simulink model "cosmic_ray_system"  (R2019a)
settings: Solver=VariableStepAuto  StartTime=0.0  StopTime=1000  RelTol=1e-3
libraries: xbsIndex_r4 x6191, casper_library_misc x163, xps_library x4, casper_library_delays x4
(part 21 of 40)

== system cosmic_ray_system/cosmic_ray/coincidence_trigger/4pt_avg/bus_addsub1 ==
  a : Inport
  b : Inport  Port=2
  a_debus : Subsystem  AncestorBlock=casper_library_flow_control/bus_expand  mask(bus_expand){mode=divisions of arbitrary size, outputNum=1, outputWidth=[24  24  24  24  24  24  24  24  24  24  24  24  24  24  24  24  24  24  24  24  24  24  24  24  24  24  24  24  24  24  24  24  24  24  24  24  24  24  24  24  24  24  24  24  24  24  24  24  24  24  24  24  24  24  24  24  24  24  24  24  24  24  24  24], outputBinaryPt=[0  0  0  0  0  0  0  0  0  0  0  0  0  0  0  0  0  0  0  0  0  0  0  0  0  0  0  0  0  0  0  0  0  0  0  0  0  0  0  0  0  0  0  0  0  0  0  0  0  0  0  0  0  0  0  0  0  0  0  0  0  0  0  0], outputArithmeticType=[1  1  1  1  1  1  1  1  1  1  1  1  1  1  1  1  1  1  1  1  1  1  1  1  1  1  1  1  1  1  1  1  1  1  1  1  1  1  1  1  1  1  1  1  1  1  1  1  1  1  1  1  1  1  1  1  1  1  1  1  1  1  1  1], show_format=on, outputToWorkspace=off, variablePrefix=, outputToModelAsWell=on}
      mask prompts: outputNum "Number of outputs:"; outputWidth "Output width [msb ... lsb]:"; outputBinaryPt "Output binary point position [msb ... lsb]:"; outputArithmeticType "Output arithmetic type (ufix=0, fix=1, bool=2) [msb ... lsb]:"; show_format "Print format string?"; outputToWorkspace "Output to workspace?"; variablePrefix "Variable name prefix:"; outputToModelAsWell "Output to model as well?"
      mask help:
      | Expands a 'bus' made using a bus_create or Xilinx
      | concat block.
      | The input will be divided into the specified number
      | of outputs with the specified arithmetic types.
      | Divisions are made from most significant bit.
      mask init: same as cosmic_ray_system/cosmic_ray/buffer_and_packetizer/bus_expand1
      settings: AttributesFormatString=64 outputs: f24.0,f24.0,f24.0,f24.0,f24.0,f24.0,f24.0,f24.0,f24.0,f24.0,f24.0,f24.0,f24.0,f24.0,f24.0,f24.0,f24.0,f24.0,f24.0,f24.0,f24.0,f24.0,f24.0,f24.0,f24.0,f24.0,f24.0,f24.0,f24.0,f24.0,f24.0,f24.0,f24.0,f24.0,f24.0,f24.0,f24.0,f24.0,f24.0,f24.0,f24.0,f24.0,f24.0,f24.0,f24.0,f24.0,f24.0,f24.0,f24.0,f24.0,f24.0,f24.0,f24.0,f24.0,f24.0,f24.0,f24.0,f24.0,f24.0,f24.0,f24.0,f24.0,f24.0,f24.0,
      mask TypeOptions mode: divisions of equal size | divisions of arbitrary size
      mask Callback mode: bus_expand_callback();
      mask Callback outputWidth: bus_expand_callback();
      mask Callback outputToWorkspace: bus_expand_callback();
  addsub{1..64} (64 alike) : xbsIndex_r4/AddSub  mode=Addition  use_carryin=off  use_carryout=off  en=off  latency=1  precision=User Defined  arith_type="Signed  (2's comp)"  n_bits=25  bin_pt=0  quantization=Truncate  overflow=Wrap  use_behavioral_HDL=on  hw_selection=Fabric  pipelined=on  dbl_ovrd=off  block_type=addsub
  b_debus : Subsystem  AncestorBlock=casper_library_flow_control/bus_expand  mask(bus_expand){mode=divisions of arbitrary size, outputNum=1, outputWidth=[24  24  24  24  24  24  24  24  24  24  24  24  24  24  24  24  24  24  24  24  24  24  24  24  24  24  24  24  24  24  24  24  24  24  24  24  24  24  24  24  24  24  24  24  24  24  24  24  24  24  24  24  24  24  24  24  24  24  24  24  24  24  24  24], outputBinaryPt=[0  0  0  0  0  0  0  0  0  0  0  0  0  0  0  0  0  0  0  0  0  0  0  0  0  0  0  0  0  0  0  0  0  0  0  0  0  0  0  0  0  0  0  0  0  0  0  0  0  0  0  0  0  0  0  0  0  0  0  0  0  0  0  0], outputArithmeticType=[1  1  1  1  1  1  1  1  1  1  1  1  1  1  1  1  1  1  1  1  1  1  1  1  1  1  1  1  1  1  1  1  1  1  1  1  1  1  1  1  1  1  1  1  1  1  1  1  1  1  1  1  1  1  1  1  1  1  1  1  1  1  1  1], show_format=on, outputToWorkspace=off, variablePrefix=, outputToModelAsWell=on}
      mask prompts: outputNum "Number of outputs:"; outputWidth "Output width [msb ... lsb]:"; outputBinaryPt "Output binary point position [msb ... lsb]:"; outputArithmeticType "Output arithmetic type (ufix=0, fix=1, bool=2) [msb ... lsb]:"; show_format "Print format string?"; outputToWorkspace "Output to workspace?"; variablePrefix "Variable name prefix:"; outputToModelAsWell "Output to model as well?"
      mask help:
      | Expands a 'bus' made using a bus_create or Xilinx
      | concat block.
      | The input will be divided into the specified number
      | of outputs with the specified arithmetic types.
      | Divisions are made from most significant bit.
      mask init: same as cosmic_ray_system/cosmic_ray/buffer_and_packetizer/bus_expand1
      settings: AttributesFormatString=64 outputs: f24.0,f24.0,f24.0,f24.0,f24.0,f24.0,f24.0,f24.0,f24.0,f24.0,f24.0,f24.0,f24.0,f24.0,f24.0,f24.0,f24.0,f24.0,f24.0,f24.0,f24.0,f24.0,f24.0,f24.0,f24.0,f24.0,f24.0,f24.0,f24.0,f24.0,f24.0,f24.0,f24.0,f24.0,f24.0,f24.0,f24.0,f24.0,f24.0,f24.0,f24.0,f24.0,f24.0,f24.0,f24.0,f24.0,f24.0,f24.0,f24.0,f24.0,f24.0,f24.0,f24.0,f24.0,f24.0,f24.0,f24.0,f24.0,f24.0,f24.0,f24.0,f24.0,f24.0,f24.0,
      mask TypeOptions mode: divisions of equal size | divisions of arbitrary size
      mask Callback mode: bus_expand_callback();
      mask Callback outputWidth: bus_expand_callback();
      mask Callback outputToWorkspace: bus_expand_callback();
  op_bussify : Subsystem  AncestorBlock=casper_library_flow_control/bus_create  mask(bus_create){inputNum=64}
      mask prompts: inputNum "Number of inputs:"
      mask init:
      | bus_create_init(gcb,...
      |     'inputNum', inputNum);
  dout : Outport
  wires:
  op_bussify/1(bus_out) -> dout/1
  addsub64/1 -> op_bussify/64(in64)
  addsub63/1 -> op_bussify/63(in63)
  addsub62/1 -> op_bussify/62(in62)
  addsub61/1 -> op_bussify/61(in61)
  addsub60/1 -> op_bussify/60(in60)
  addsub59/1 -> op_bussify/59(in59)
  addsub58/1 -> op_bussify/58(in58)
  addsub57/1 -> op_bussify/57(in57)
  addsub56/1 -> op_bussify/56(in56)
  addsub55/1 -> op_bussify/55(in55)
  addsub54/1 -> op_bussify/54(in54)
  addsub53/1 -> op_bussify/53(in53)
  addsub52/1 -> op_bussify/52(in52)
  addsub51/1 -> op_bussify/51(in51)
  addsub50/1 -> op_bussify/50(in50)
  addsub49/1 -> op_bussify/49(in49)
  addsub48/1 -> op_bussify/48(in48)
  addsub47/1 -> op_bussify/47(in47)
  addsub46/1 -> op_bussify/46(in46)
  addsub45/1 -> op_bussify/45(in45)
  addsub44/1 -> op_bussify/44(in44)
  addsub43/1 -> op_bussify/43(in43)
  addsub42/1 -> op_bussify/42(in42)
  addsub41/1 -> op_bussify/41(in41)
  addsub40/1 -> op_bussify/40(in40)
  addsub39/1 -> op_bussify/39(in39)
  addsub38/1 -> op_bussify/38(in38)
  addsub37/1 -> op_bussify/37(in37)
  addsub36/1 -> op_bussify/36(in36)
  addsub35/1 -> op_bussify/35(in35)
  addsub34/1 -> op_bussify/34(in34)
  addsub33/1 -> op_bussify/33(in33)
  addsub32/1 -> op_bussify/32(in32)
  addsub31/1 -> op_bussify/31(in31)
  addsub30/1 -> op_bussify/30(in30)
  addsub29/1 -> op_bussify/29(in29)
  addsub28/1 -> op_bussify/28(in28)
  addsub27/1 -> op_bussify/27(in27)
  addsub26/1 -> op_bussify/26(in26)
  addsub25/1 -> op_bussify/25(in25)
  addsub24/1 -> op_bussify/24(in24)
  addsub23/1 -> op_bussify/23(in23)
  addsub22/1 -> op_bussify/22(in22)
  addsub21/1 -> op_bussify/21(in21)
  addsub20/1 -> op_bussify/20(in20)
  addsub19/1 -> op_bussify/19(in19)
  addsub18/1 -> op_bussify/18(in18)
  addsub17/1 -> op_bussify/17(in17)
  addsub16/1 -> op_bussify/16(in16)
  addsub15/1 -> op_bussify/15(in15)
  addsub14/1 -> op_bussify/14(in14)
  addsub13/1 -> op_bussify/13(in13)
  addsub12/1 -> op_bussify/12(in12)
  addsub11/1 -> op_bussify/11(in11)
  addsub10/1 -> op_bussify/10(in10)
  addsub9/1 -> op_bussify/9(in9)
  addsub8/1 -> op_bussify/8(in8)
  addsub7/1 -> op_bussify/7(in7)
  addsub6/1 -> op_bussify/6(in6)
  addsub5/1 -> op_bussify/5(in5)
  addsub4/1 -> op_bussify/4(in4)
  addsub3/1 -> op_bussify/3(in3)
  addsub2/1 -> op_bussify/2(in2)
  addsub1/1 -> op_bussify/1(in1)
  b_debus/64(lsb_out1) -> addsub64/2
  a_debus/64(lsb_out1) -> addsub64/1
  b_debus/63(out2) -> addsub63/2
  a_debus/63(out2) -> addsub63/1
  b_debus/62(out3) -> addsub62/2
  a_debus/62(out3) -> addsub62/1
  b_debus/61(out4) -> addsub61/2
  a_debus/61(out4) -> addsub61/1
  b_debus/60(out5) -> addsub60/2
  a_debus/60(out5) -> addsub60/1
  b_debus/59(out6) -> addsub59/2
  a_debus/59(out6) -> addsub59/1
  b_debus/58(out7) -> addsub58/2
  a_debus/58(out7) -> addsub58/1
  b_debus/57(out8) -> addsub57/2
  a_debus/57(out8) -> addsub57/1
  b_debus/56(out9) -> addsub56/2
  a_debus/56(out9) -> addsub56/1
  b_debus/55(out10) -> addsub55/2
  a_debus/55(out10) -> addsub55/1
  b_debus/54(out11) -> addsub54/2
  a_debus/54(out11) -> addsub54/1
  b_debus/53(out12) -> addsub53/2
  a_debus/53(out12) -> addsub53/1
  b_debus/52(out13) -> addsub52/2
  a_debus/52(out13) -> addsub52/1
  b_debus/51(out14) -> addsub51/2
  a_debus/51(out14) -> addsub51/1
  b_debus/50(out15) -> addsub50/2
  a_debus/50(out15) -> addsub50/1
  b_debus/49(out16) -> addsub49/2
  a_debus/49(out16) -> addsub49/1
  b_debus/48(out17) -> addsub48/2
  a_debus/48(out17) -> addsub48/1
  b_debus/47(out18) -> addsub47/2
  a_debus/47(out18) -> addsub47/1
  b_debus/46(out19) -> addsub46/2
  a_debus/46(out19) -> addsub46/1
  b_debus/45(out20) -> addsub45/2
  a_debus/45(out20) -> addsub45/1
  b_debus/44(out21) -> addsub44/2
  a_debus/44(out21) -> addsub44/1
  b_debus/43(out22) -> addsub43/2
  a_debus/43(out22) -> addsub43/1
  b_debus/42(out23) -> addsub42/2
  a_debus/42(out23) -> addsub42/1
  b_debus/41(out24) -> addsub41/2
  a_debus/41(out24) -> addsub41/1
  b_debus/40(out25) -> addsub40/2
  a_debus/40(out25) -> addsub40/1
  b_debus/39(out26) -> addsub39/2
  a_debus/39(out26) -> addsub39/1
  b_debus/38(out27) -> addsub38/2
  a_debus/38(out27) -> addsub38/1
  b_debus/37(out28) -> addsub37/2
  a_debus/37(out28) -> addsub37/1
  b_debus/36(out29) -> addsub36/2
  a_debus/36(out29) -> addsub36/1
  b_debus/35(out30) -> addsub35/2
  a_debus/35(out30) -> addsub35/1
  b_debus/34(out31) -> addsub34/2
  a_debus/34(out31) -> addsub34/1
  b_debus/33(out32) -> addsub33/2
  a_debus/33(out32) -> addsub33/1
  b_debus/32(out33) -> addsub32/2
  a_debus/32(out33) -> addsub32/1
  b_debus/31(out34) -> addsub31/2
  a_debus/31(out34) -> addsub31/1
  b_debus/30(out35) -> addsub30/2
  a_debus/30(out35) -> addsub30/1
  b_debus/29(out36) -> addsub29/2
  a_debus/29(out36) -> addsub29/1
  b_debus/28(out37) -> addsub28/2
  a_debus/28(out37) -> addsub28/1
  b_debus/27(out38) -> addsub27/2
  a_debus/27(out38) -> addsub27/1
  b_debus/26(out39) -> addsub26/2
  a_debus/26(out39) -> addsub26/1
  b_debus/25(out40) -> addsub25/2
  a_debus/25(out40) -> addsub25/1
  b_debus/24(out41) -> addsub24/2
  a_debus/24(out41) -> addsub24/1
  b_debus/23(out42) -> addsub23/2
  a_debus/23(out42) -> addsub23/1
  b_debus/22(out43) -> addsub22/2
  a_debus/22(out43) -> addsub22/1
  b_debus/21(out44) -> addsub21/2
  a_debus/21(out44) -> addsub21/1
  b_debus/20(out45) -> addsub20/2
  a_debus/20(out45) -> addsub20/1
  b_debus/19(out46) -> addsub19/2
  a_debus/19(out46) -> addsub19/1
  b_debus/18(out47) -> addsub18/2
  a_debus/18(out47) -> addsub18/1
  b_debus/17(out48) -> addsub17/2
  a_debus/17(out48) -> addsub17/1
  b_debus/16(out49) -> addsub16/2
  a_debus/16(out49) -> addsub16/1
  b_debus/15(out50) -> addsub15/2
  a_debus/15(out50) -> addsub15/1
  b_debus/14(out51) -> addsub14/2
  a_debus/14(out51) -> addsub14/1
  b_debus/13(out52) -> addsub13/2
  a_debus/13(out52) -> addsub13/1
  b_debus/12(out53) -> addsub12/2
  a_debus/12(out53) -> addsub12/1
  b_debus/11(out54) -> addsub11/2
  a_debus/11(out54) -> addsub11/1
  b_debus/10(out55) -> addsub10/2
  a_debus/10(out55) -> addsub10/1
  b_debus/9(out56) -> addsub9/2
  a_debus/9(out56) -> addsub9/1
  b_debus/8(out57) -> addsub8/2
  a_debus/8(out57) -> addsub8/1
  b_debus/7(out58) -> addsub7/2
  a_debus/7(out58) -> addsub7/1
  b_debus/6(out59) -> addsub6/2
  a_debus/6(out59) -> addsub6/1
  b_debus/5(out60) -> addsub5/2
  a_debus/5(out60) -> addsub5/1
  b_debus/4(out61) -> addsub4/2
  a_debus/4(out61) -> addsub4/1
  b_debus/3(out62) -> addsub3/2
  a_debus/3(out62) -> addsub3/1
  b_debus/2(out63) -> addsub2/2
  a_debus/2(out63) -> addsub2/1
  b_debus/1(msb_out64) -> addsub1/2
  a_debus/1(msb_out64) -> addsub1/1
  b/1 -> b_debus/1(bus_in)
  a/1 -> a_debus/1(bus_in)

== system cosmic_ray_system/cosmic_ray/coincidence_trigger/4pt_avg/bus_addsub2 ==
  a : Inport
  b : Inport  Port=2
  a_debus : Subsystem  AncestorBlock=casper_library_flow_control/bus_expand  mask(bus_expand){mode=divisions of arbitrary size, outputNum=1, outputWidth=[25  25  25  25  25  25  25  25  25  25  25  25  25  25  25  25  25  25  25  25  25  25  25  25  25  25  25  25  25  25  25  25  25  25  25  25  25  25  25  25  25  25  25  25  25  25  25  25  25  25  25  25  25  25  25  25  25  25  25  25  25  25  25  25], outputBinaryPt=[0  0  0  0  0  0  0  0  0  0  0  0  0  0  0  0  0  0  0  0  0  0  0  0  0  0  0  0  0  0  0  0  0  0  0  0  0  0  0  0  0  0  0  0  0  0  0  0  0  0  0  0  0  0  0  0  0  0  0  0  0  0  0  0], outputArithmeticType=[1  1  1  1  1  1  1  1  1  1  1  1  1  1  1  1  1  1  1  1  1  1  1  1  1  1  1  1  1  1  1  1  1  1  1  1  1  1  1  1  1  1  1  1  1  1  1  1  1  1  1  1  1  1  1  1  1  1  1  1  1  1  1  1], show_format=on, outputToWorkspace=off, variablePrefix=, outputToModelAsWell=on}
      mask prompts: outputNum "Number of outputs:"; outputWidth "Output width [msb ... lsb]:"; outputBinaryPt "Output binary point position [msb ... lsb]:"; outputArithmeticType "Output arithmetic type (ufix=0, fix=1, bool=2) [msb ... lsb]:"; show_format "Print format string?"; outputToWorkspace "Output to workspace?"; variablePrefix "Variable name prefix:"; outputToModelAsWell "Output to model as well?"
      mask help:
      | Expands a 'bus' made using a bus_create or Xilinx
      | concat block.
      | The input will be divided into the specified number
      | of outputs with the specified arithmetic types.
      | Divisions are made from most significant bit.
      mask init: same as cosmic_ray_system/cosmic_ray/buffer_and_packetizer/bus_expand1
      settings: AttributesFormatString=64 outputs: f25.0,f25.0,f25.0,f25.0,f25.0,f25.0,f25.0,f25.0,f25.0,f25.0,f25.0,f25.0,f25.0,f25.0,f25.0,f25.0,f25.0,f25.0,f25.0,f25.0,f25.0,f25.0,f25.0,f25.0,f25.0,f25.0,f25.0,f25.0,f25.0,f25.0,f25.0,f25.0,f25.0,f25.0,f25.0,f25.0,f25.0,f25.0,f25.0,f25.0,f25.0,f25.0,f25.0,f25.0,f25.0,f25.0,f25.0,f25.0,f25.0,f25.0,f25.0,f25.0,f25.0,f25.0,f25.0,f25.0,f25.0,f25.0,f25.0,f25.0,f25.0,f25.0,f25.0,f25.0,
      mask TypeOptions mode: divisions of equal size | divisions of arbitrary size
      mask Callback mode: bus_expand_callback();
      mask Callback outputWidth: bus_expand_callback();
      mask Callback outputToWorkspace: bus_expand_callback();
  addsub{1..64} (64 alike) : xbsIndex_r4/AddSub  mode=Addition  use_carryin=off  use_carryout=off  en=off  latency=1  precision=User Defined  arith_type="Signed  (2's comp)"  n_bits=26  bin_pt=0  quantization=Truncate  overflow=Wrap  use_behavioral_HDL=on  hw_selection=Fabric  pipelined=on  dbl_ovrd=off  block_type=addsub
  b_debus : Subsystem  AncestorBlock=casper_library_flow_control/bus_expand  mask(bus_expand){mode=divisions of arbitrary size, outputNum=1, outputWidth=[25  25  25  25  25  25  25  25  25  25  25  25  25  25  25  25  25  25  25  25  25  25  25  25  25  25  25  25  25  25  25  25  25  25  25  25  25  25  25  25  25  25  25  25  25  25  25  25  25  25  25  25  25  25  25  25  25  25  25  25  25  25  25  25], outputBinaryPt=[0  0  0  0  0  0  0  0  0  0  0  0  0  0  0  0  0  0  0  0  0  0  0  0  0  0  0  0  0  0  0  0  0  0  0  0  0  0  0  0  0  0  0  0  0  0  0  0  0  0  0  0  0  0  0  0  0  0  0  0  0  0  0  0], outputArithmeticType=[1  1  1  1  1  1  1  1  1  1  1  1  1  1  1  1  1  1  1  1  1  1  1  1  1  1  1  1  1  1  1  1  1  1  1  1  1  1  1  1  1  1  1  1  1  1  1  1  1  1  1  1  1  1  1  1  1  1  1  1  1  1  1  1], show_format=on, outputToWorkspace=off, variablePrefix=, outputToModelAsWell=on}
      mask prompts: outputNum "Number of outputs:"; outputWidth "Output width [msb ... lsb]:"; outputBinaryPt "Output binary point position [msb ... lsb]:"; outputArithmeticType "Output arithmetic type (ufix=0, fix=1, bool=2) [msb ... lsb]:"; show_format "Print format string?"; outputToWorkspace "Output to workspace?"; variablePrefix "Variable name prefix:"; outputToModelAsWell "Output to model as well?"
      mask help:
      | Expands a 'bus' made using a bus_create or Xilinx
      | concat block.
      | The input will be divided into the specified number
      | of outputs with the specified arithmetic types.
      | Divisions are made from most significant bit.
      mask init: same as cosmic_ray_system/cosmic_ray/buffer_and_packetizer/bus_expand1
      settings: AttributesFormatString=64 outputs: f25.0,f25.0,f25.0,f25.0,f25.0,f25.0,f25.0,f25.0,f25.0,f25.0,f25.0,f25.0,f25.0,f25.0,f25.0,f25.0,f25.0,f25.0,f25.0,f25.0,f25.0,f25.0,f25.0,f25.0,f25.0,f25.0,f25.0,f25.0,f25.0,f25.0,f25.0,f25.0,f25.0,f25.0,f25.0,f25.0,f25.0,f25.0,f25.0,f25.0,f25.0,f25.0,f25.0,f25.0,f25.0,f25.0,f25.0,f25.0,f25.0,f25.0,f25.0,f25.0,f25.0,f25.0,f25.0,f25.0,f25.0,f25.0,f25.0,f25.0,f25.0,f25.0,f25.0,f25.0,
      mask TypeOptions mode: divisions of equal size | divisions of arbitrary size
      mask Callback mode: bus_expand_callback();
      mask Callback outputWidth: bus_expand_callback();
      mask Callback outputToWorkspace: bus_expand_callback();
  op_bussify : Subsystem  AncestorBlock=casper_library_flow_control/bus_create  mask(bus_create){inputNum=64}
      mask prompts: inputNum "Number of inputs:"
      mask init:
      | bus_create_init(gcb,...
      |     'inputNum', inputNum);
  dout : Outport
  wires:
  a/1 -> a_debus/1(bus_in)
  b/1 -> b_debus/1(bus_in)
  a_debus/1(msb_out64) -> addsub1/1
  b_debus/1(msb_out64) -> addsub1/2
  a_debus/2(out63) -> addsub2/1
  b_debus/2(out63) -> addsub2/2
  a_debus/3(out62) -> addsub3/1
  b_debus/3(out62) -> addsub3/2
  a_debus/4(out61) -> addsub4/1
  b_debus/4(out61) -> addsub4/2
  a_debus/5(out60) -> addsub5/1
  b_debus/5(out60) -> addsub5/2
  a_debus/6(out59) -> addsub6/1
  b_debus/6(out59) -> addsub6/2
  a_debus/7(out58) -> addsub7/1
  b_debus/7(out58) -> addsub7/2
  a_debus/8(out57) -> addsub8/1
  b_debus/8(out57) -> addsub8/2
  a_debus/9(out56) -> addsub9/1
  b_debus/9(out56) -> addsub9/2
  a_debus/10(out55) -> addsub10/1
  b_debus/10(out55) -> addsub10/2
  a_debus/11(out54) -> addsub11/1
  b_debus/11(out54) -> addsub11/2
  a_debus/12(out53) -> addsub12/1
  b_debus/12(out53) -> addsub12/2
  a_debus/13(out52) -> addsub13/1
  b_debus/13(out52) -> addsub13/2
  a_debus/14(out51) -> addsub14/1
  b_debus/14(out51) -> addsub14/2
  a_debus/15(out50) -> addsub15/1
  b_debus/15(out50) -> addsub15/2
  a_debus/16(out49) -> addsub16/1
  b_debus/16(out49) -> addsub16/2
  a_debus/17(out48) -> addsub17/1
  b_debus/17(out48) -> addsub17/2
  a_debus/18(out47) -> addsub18/1
  b_debus/18(out47) -> addsub18/2
  a_debus/19(out46) -> addsub19/1
  b_debus/19(out46) -> addsub19/2
  a_debus/20(out45) -> addsub20/1
  b_debus/20(out45) -> addsub20/2
  a_debus/21(out44) -> addsub21/1
  b_debus/21(out44) -> addsub21/2
  a_debus/22(out43) -> addsub22/1
  b_debus/22(out43) -> addsub22/2
  a_debus/23(out42) -> addsub23/1
  b_debus/23(out42) -> addsub23/2
  a_debus/24(out41) -> addsub24/1
  b_debus/24(out41) -> addsub24/2
  a_debus/25(out40) -> addsub25/1
  b_debus/25(out40) -> addsub25/2
  a_debus/26(out39) -> addsub26/1
  b_debus/26(out39) -> addsub26/2
  a_debus/27(out38) -> addsub27/1
  b_debus/27(out38) -> addsub27/2
  a_debus/28(out37) -> addsub28/1
  b_debus/28(out37) -> addsub28/2
  a_debus/29(out36) -> addsub29/1
  b_debus/29(out36) -> addsub29/2
  a_debus/30(out35) -> addsub30/1
  b_debus/30(out35) -> addsub30/2
  a_debus/31(out34) -> addsub31/1
  b_debus/31(out34) -> addsub31/2
  a_debus/32(out33) -> addsub32/1
  b_debus/32(out33) -> addsub32/2
  a_debus/33(out32) -> addsub33/1
  b_debus/33(out32) -> addsub33/2
  a_debus/34(out31) -> addsub34/1
  b_debus/34(out31) -> addsub34/2
  a_debus/35(out30) -> addsub35/1
  b_debus/35(out30) -> addsub35/2
  a_debus/36(out29) -> addsub36/1
  b_debus/36(out29) -> addsub36/2
  a_debus/37(out28) -> addsub37/1
  b_debus/37(out28) -> addsub37/2
  a_debus/38(out27) -> addsub38/1
  b_debus/38(out27) -> addsub38/2
  a_debus/39(out26) -> addsub39/1
  b_debus/39(out26) -> addsub39/2
  a_debus/40(out25) -> addsub40/1
  b_debus/40(out25) -> addsub40/2
  a_debus/41(out24) -> addsub41/1
  b_debus/41(out24) -> addsub41/2
  a_debus/42(out23) -> addsub42/1
  b_debus/42(out23) -> addsub42/2
  a_debus/43(out22) -> addsub43/1
  b_debus/43(out22) -> addsub43/2
  a_debus/44(out21) -> addsub44/1
  b_debus/44(out21) -> addsub44/2
  a_debus/45(out20) -> addsub45/1
  b_debus/45(out20) -> addsub45/2
  a_debus/46(out19) -> addsub46/1
  b_debus/46(out19) -> addsub46/2
  a_debus/47(out18) -> addsub47/1
  b_debus/47(out18) -> addsub47/2
  a_debus/48(out17) -> addsub48/1
  b_debus/48(out17) -> addsub48/2
  a_debus/49(out16) -> addsub49/1
  b_debus/49(out16) -> addsub49/2
  a_debus/50(out15) -> addsub50/1
  b_debus/50(out15) -> addsub50/2
  a_debus/51(out14) -> addsub51/1
  b_debus/51(out14) -> addsub51/2
  a_debus/52(out13) -> addsub52/1
  b_debus/52(out13) -> addsub52/2
  a_debus/53(out12) -> addsub53/1
  b_debus/53(out12) -> addsub53/2
  a_debus/54(out11) -> addsub54/1
  b_debus/54(out11) -> addsub54/2
  a_debus/55(out10) -> addsub55/1
  b_debus/55(out10) -> addsub55/2
  a_debus/56(out9) -> addsub56/1
  b_debus/56(out9) -> addsub56/2
  a_debus/57(out8) -> addsub57/1
  b_debus/57(out8) -> addsub57/2
  a_debus/58(out7) -> addsub58/1
  b_debus/58(out7) -> addsub58/2
  a_debus/59(out6) -> addsub59/1
  b_debus/59(out6) -> addsub59/2
  a_debus/60(out5) -> addsub60/1
  b_debus/60(out5) -> addsub60/2
  a_debus/61(out4) -> addsub61/1
  b_debus/61(out4) -> addsub61/2
  a_debus/62(out3) -> addsub62/1
  b_debus/62(out3) -> addsub62/2
  a_debus/63(out2) -> addsub63/1
  b_debus/63(out2) -> addsub63/2
  a_debus/64(lsb_out1) -> addsub64/1
  b_debus/64(lsb_out1) -> addsub64/2
  addsub1/1 -> op_bussify/1(in1)
  addsub2/1 -> op_bussify/2(in2)
  addsub3/1 -> op_bussify/3(in3)
  addsub4/1 -> op_bussify/4(in4)
  addsub5/1 -> op_bussify/5(in5)
  addsub6/1 -> op_bussify/6(in6)
  addsub7/1 -> op_bussify/7(in7)
  addsub8/1 -> op_bussify/8(in8)
  addsub9/1 -> op_bussify/9(in9)
  addsub10/1 -> op_bussify/10(in10)
  addsub11/1 -> op_bussify/11(in11)
  addsub12/1 -> op_bussify/12(in12)
  addsub13/1 -> op_bussify/13(in13)
  addsub14/1 -> op_bussify/14(in14)
  addsub15/1 -> op_bussify/15(in15)
  addsub16/1 -> op_bussify/16(in16)
  addsub17/1 -> op_bussify/17(in17)
  addsub18/1 -> op_bussify/18(in18)
  addsub19/1 -> op_bussify/19(in19)
  addsub20/1 -> op_bussify/20(in20)
  addsub21/1 -> op_bussify/21(in21)
  addsub22/1 -> op_bussify/22(in22)
  addsub23/1 -> op_bussify/23(in23)
  addsub24/1 -> op_bussify/24(in24)
  addsub25/1 -> op_bussify/25(in25)
  addsub26/1 -> op_bussify/26(in26)
  addsub27/1 -> op_bussify/27(in27)
  addsub28/1 -> op_bussify/28(in28)
  addsub29/1 -> op_bussify/29(in29)
  addsub30/1 -> op_bussify/30(in30)
  addsub31/1 -> op_bussify/31(in31)
  addsub32/1 -> op_bussify/32(in32)
  addsub33/1 -> op_bussify/33(in33)
  addsub34/1 -> op_bussify/34(in34)
  addsub35/1 -> op_bussify/35(in35)
  addsub36/1 -> op_bussify/36(in36)
  addsub37/1 -> op_bussify/37(in37)
  addsub38/1 -> op_bussify/38(in38)
  addsub39/1 -> op_bussify/39(in39)
  addsub40/1 -> op_bussify/40(in40)
  addsub41/1 -> op_bussify/41(in41)
  addsub42/1 -> op_bussify/42(in42)
  addsub43/1 -> op_bussify/43(in43)
  addsub44/1 -> op_bussify/44(in44)
  addsub45/1 -> op_bussify/45(in45)
  addsub46/1 -> op_bussify/46(in46)
  addsub47/1 -> op_bussify/47(in47)
  addsub48/1 -> op_bussify/48(in48)
  addsub49/1 -> op_bussify/49(in49)
  addsub50/1 -> op_bussify/50(in50)
  addsub51/1 -> op_bussify/51(in51)
  addsub52/1 -> op_bussify/52(in52)
  addsub53/1 -> op_bussify/53(in53)
  addsub54/1 -> op_bussify/54(in54)
  addsub55/1 -> op_bussify/55(in55)
  addsub56/1 -> op_bussify/56(in56)
  addsub57/1 -> op_bussify/57(in57)
  addsub58/1 -> op_bussify/58(in58)
  addsub59/1 -> op_bussify/59(in59)
  addsub60/1 -> op_bussify/60(in60)
  addsub61/1 -> op_bussify/61(in61)
  addsub62/1 -> op_bussify/62(in62)
  addsub63/1 -> op_bussify/63(in63)
  addsub64/1 -> op_bussify/64(in64)
  op_bussify/1(bus_out) -> dout/1

== system cosmic_ray_system/cosmic_ray/coincidence_trigger/FIR1/bus_create2 ==
  in1 : Inport
  in2 : Inport  Port=2
  in3 : Inport  Port=3
  in4 : Inport  Port=4
  in5 : Inport  Port=5
  in6 : Inport  Port=6
  in7 : Inport  Port=7
  in8 : Inport  Port=8
  in9 : Inport  Port=9
  in10 : Inport  Port=10
  in11 : Inport  Port=11
  in12 : Inport  Port=12
  in13 : Inport  Port=13
  in14 : Inport  Port=14
  in15 : Inport  Port=15
  in16 : Inport  Port=16
  in17 : Inport  Port=17
  in18 : Inport  Port=18
  in19 : Inport  Port=19
  in20 : Inport  Port=20
  in21 : Inport  Port=21
  in22 : Inport  Port=22
  in23 : Inport  Port=23
  in24 : Inport  Port=24
  in25 : Inport  Port=25
  in26 : Inport  Port=26
  in27 : Inport  Port=27
  in28 : Inport  Port=28
  in29 : Inport  Port=29
  in30 : Inport  Port=30
  in31 : Inport  Port=31
  in32 : Inport  Port=32
  in33 : Inport  Port=33
  in34 : Inport  Port=34
  in35 : Inport  Port=35
  in36 : Inport  Port=36
  in37 : Inport  Port=37
  in38 : Inport  Port=38
  in39 : Inport  Port=39
  in40 : Inport  Port=40
  in41 : Inport  Port=41
  in42 : Inport  Port=42
  in43 : Inport  Port=43
  in44 : Inport  Port=44
  in45 : Inport  Port=45
  in46 : Inport  Port=46
  in47 : Inport  Port=47
  in48 : Inport  Port=48
  in49 : Inport  Port=49
  in50 : Inport  Port=50
  in51 : Inport  Port=51
  in52 : Inport  Port=52
  in53 : Inport  Port=53
  in54 : Inport  Port=54
  in55 : Inport  Port=55
  in56 : Inport  Port=56
  in57 : Inport  Port=57
  in58 : Inport  Port=58
  in59 : Inport  Port=59
  in60 : Inport  Port=60
  in61 : Inport  Port=61
  in62 : Inport  Port=62
  in63 : Inport  Port=63
  in64 : Inport  Port=64
  concatenate : xbsIndex_r4/Concat  num_inputs=64  dbl_ovrd=off  block_type=concat
  reinterpret{1..64} (64 alike) : xbsIndex_r4/Reinterpret  force_arith_type=on  arith_type=Unsigned  force_bin_pt=on  bin_pt=0  block_type=reinterpret
      reinterpret1 settings: infoedit="Changes signal type without altering the binary representation.   You can changed the signal between signed and unsigned, and relocate the binary point.<br><br>Hardware notes: In hardware this block costs nothing.<br><br>Example:  Suppose the input is 6 bits wide, signed, with 2 fractional bits, and the output is forced to unsigned with 0 fractional bits.  Then an input of -2.0 (1110.00 in binary 2's complement) becomes an output of 56 (111000 in binary)."
      reinterpret2 settings: infoedit="Changes signal type without altering the binary representation.   You can changed the signal between signed and unsigned, and relocate the binary point.<br><br>Hardware notes: In hardware this block costs nothing.<br><br>Example:  Suppose the input is 6 bits wide, signed, with 2 fractional bits, and the output is forced to unsigned with 0 fractional bits.  Then an input of -2.0 (1110.00 in binary 2's complement) becomes an output of 56 (111000 in binary)."
  bus_out : Outport
  wires:
  concatenate/1 -> bus_out/1
  in1/1 -> reinterpret1/1
  reinterpret1/1 -> concatenate/1
  in2/1 -> reinterpret2/1
  reinterpret2/1 -> concatenate/2
  in3/1 -> reinterpret3/1
  reinterpret3/1 -> concatenate/3
  in4/1 -> reinterpret4/1
  reinterpret4/1 -> concatenate/4
  in5/1 -> reinterpret5/1
  reinterpret5/1 -> concatenate/5
  in6/1 -> reinterpret6/1
  reinterpret6/1 -> concatenate/6
  in7/1 -> reinterpret7/1
  reinterpret7/1 -> concatenate/7
  in8/1 -> reinterpret8/1
  reinterpret8/1 -> concatenate/8
  in9/1 -> reinterpret9/1
  reinterpret9/1 -> concatenate/9
  in10/1 -> reinterpret10/1
  reinterpret10/1 -> concatenate/10
  in11/1 -> reinterpret11/1
  reinterpret11/1 -> concatenate/11
  in12/1 -> reinterpret12/1
  reinterpret12/1 -> concatenate/12
  in13/1 -> reinterpret13/1
  reinterpret13/1 -> concatenate/13
  in14/1 -> reinterpret14/1
  reinterpret14/1 -> concatenate/14
  in15/1 -> reinterpret15/1
  reinterpret15/1 -> concatenate/15
  in16/1 -> reinterpret16/1
  reinterpret16/1 -> concatenate/16
  in17/1 -> reinterpret17/1
  reinterpret17/1 -> concatenate/17
  in18/1 -> reinterpret18/1
  reinterpret18/1 -> concatenate/18
  in19/1 -> reinterpret19/1
  reinterpret19/1 -> concatenate/19
  in20/1 -> reinterpret20/1
  reinterpret20/1 -> concatenate/20
  in21/1 -> reinterpret21/1
  reinterpret21/1 -> concatenate/21
  in22/1 -> reinterpret22/1
  reinterpret22/1 -> concatenate/22
  in23/1 -> reinterpret23/1
  reinterpret23/1 -> concatenate/23
  in24/1 -> reinterpret24/1
  reinterpret24/1 -> concatenate/24
  in25/1 -> reinterpret25/1
  reinterpret25/1 -> concatenate/25
  in26/1 -> reinterpret26/1
  reinterpret26/1 -> concatenate/26
  in27/1 -> reinterpret27/1
  reinterpret27/1 -> concatenate/27
  in28/1 -> reinterpret28/1
  reinterpret28/1 -> concatenate/28
  in29/1 -> reinterpret29/1
  reinterpret29/1 -> concatenate/29
  in30/1 -> reinterpret30/1
  reinterpret30/1 -> concatenate/30
  in31/1 -> reinterpret31/1
  reinterpret31/1 -> concatenate/31
  in32/1 -> reinterpret32/1
  reinterpret32/1 -> concatenate/32
  in33/1 -> reinterpret33/1
  reinterpret33/1 -> concatenate/33
  in34/1 -> reinterpret34/1
  reinterpret34/1 -> concatenate/34
  in35/1 -> reinterpret35/1
  reinterpret35/1 -> concatenate/35
  in36/1 -> reinterpret36/1
  reinterpret36/1 -> concatenate/36
  in37/1 -> reinterpret37/1
  reinterpret37/1 -> concatenate/37
  in38/1 -> reinterpret38/1
  reinterpret38/1 -> concatenate/38
  in39/1 -> reinterpret39/1
  reinterpret39/1 -> concatenate/39
  in40/1 -> reinterpret40/1
  reinterpret40/1 -> concatenate/40
  in41/1 -> reinterpret41/1
  reinterpret41/1 -> concatenate/41
  in42/1 -> reinterpret42/1
  reinterpret42/1 -> concatenate/42
  in43/1 -> reinterpret43/1
  reinterpret43/1 -> concatenate/43
  in44/1 -> reinterpret44/1
  reinterpret44/1 -> concatenate/44
  in45/1 -> reinterpret45/1
  reinterpret45/1 -> concatenate/45
  in46/1 -> reinterpret46/1
  reinterpret46/1 -> concatenate/46
  in47/1 -> reinterpret47/1
  reinterpret47/1 -> concatenate/47
  in48/1 -> reinterpret48/1
  reinterpret48/1 -> concatenate/48
  in49/1 -> reinterpret49/1
  reinterpret49/1 -> concatenate/49
  in50/1 -> reinterpret50/1
  reinterpret50/1 -> concatenate/50
  in51/1 -> reinterpret51/1
  reinterpret51/1 -> concatenate/51
  in52/1 -> reinterpret52/1
  reinterpret52/1 -> concatenate/52
  in53/1 -> reinterpret53/1
  reinterpret53/1 -> concatenate/53
  in54/1 -> reinterpret54/1
  reinterpret54/1 -> concatenate/54
  in55/1 -> reinterpret55/1
  reinterpret55/1 -> concatenate/55
  in56/1 -> reinterpret56/1
  reinterpret56/1 -> concatenate/56
  in57/1 -> reinterpret57/1
  reinterpret57/1 -> concatenate/57
  in58/1 -> reinterpret58/1
  reinterpret58/1 -> concatenate/58
  in59/1 -> reinterpret59/1
  reinterpret59/1 -> concatenate/59
  in60/1 -> reinterpret60/1
  reinterpret60/1 -> concatenate/60
  in61/1 -> reinterpret61/1
  reinterpret61/1 -> concatenate/61
  in62/1 -> reinterpret62/1
  reinterpret62/1 -> concatenate/62
  in63/1 -> reinterpret63/1
  reinterpret63/1 -> concatenate/63
  in64/1 -> reinterpret64/1
  reinterpret64/1 -> concatenate/64

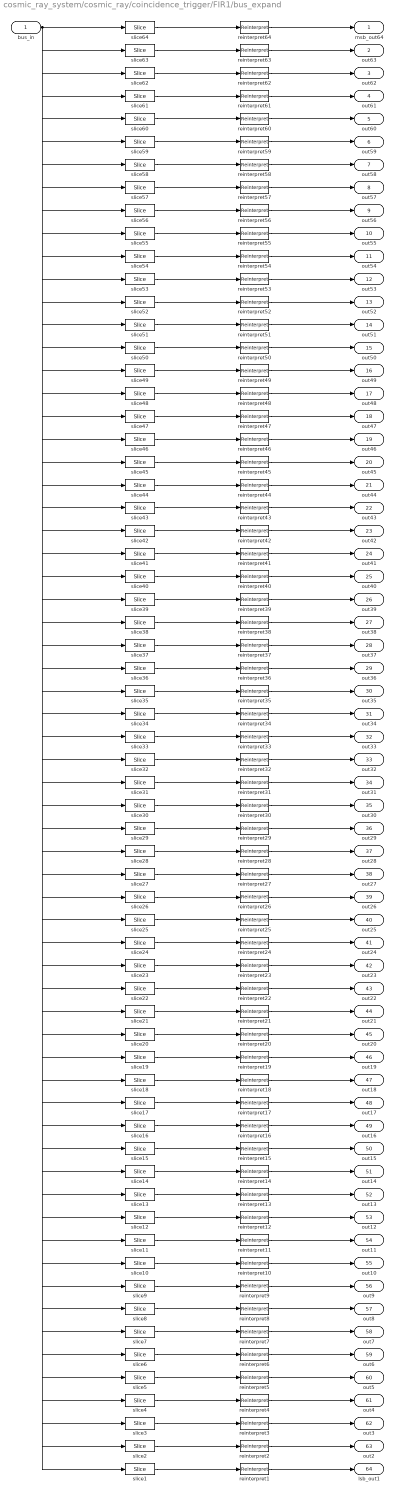
== system cosmic_ray_system/cosmic_ray/coincidence_trigger/FIR1/bus_expand ==
  bus_in : Inport
  reinterpret{1..64} (64 alike) : xbsIndex_r4/Reinterpret  force_arith_type=on  arith_type="Signed  (2's comp)"  force_bin_pt=on  bin_pt=0  block_type=reinterpret
  slice1 : xbsIndex_r4/Slice  nbits=10  boolean_output=off  mode=Upper Bit Location + Width  bit1=-630  base1=MSB of Input  bit0=0  base0=LSB of Input  dbl_ovrd=off  block_type=slice
  slice10 : xbsIndex_r4/Slice  nbits=10  boolean_output=off  mode=Upper Bit Location + Width  bit1=-540  base1=MSB of Input  bit0=0  base0=LSB of Input  dbl_ovrd=off  block_type=slice
  slice11 : xbsIndex_r4/Slice  nbits=10  boolean_output=off  mode=Upper Bit Location + Width  bit1=-530  base1=MSB of Input  bit0=0  base0=LSB of Input  dbl_ovrd=off  block_type=slice
  slice12 : xbsIndex_r4/Slice  nbits=10  boolean_output=off  mode=Upper Bit Location + Width  bit1=-520  base1=MSB of Input  bit0=0  base0=LSB of Input  dbl_ovrd=off  block_type=slice
  slice13 : xbsIndex_r4/Slice  nbits=10  boolean_output=off  mode=Upper Bit Location + Width  bit1=-510  base1=MSB of Input  bit0=0  base0=LSB of Input  dbl_ovrd=off  block_type=slice
  slice14 : xbsIndex_r4/Slice  nbits=10  boolean_output=off  mode=Upper Bit Location + Width  bit1=-500  base1=MSB of Input  bit0=0  base0=LSB of Input  dbl_ovrd=off  block_type=slice
  slice15 : xbsIndex_r4/Slice  nbits=10  boolean_output=off  mode=Upper Bit Location + Width  bit1=-490  base1=MSB of Input  bit0=0  base0=LSB of Input  dbl_ovrd=off  block_type=slice
  slice16 : xbsIndex_r4/Slice  nbits=10  boolean_output=off  mode=Upper Bit Location + Width  bit1=-480  base1=MSB of Input  bit0=0  base0=LSB of Input  dbl_ovrd=off  block_type=slice
  slice17 : xbsIndex_r4/Slice  nbits=10  boolean_output=off  mode=Upper Bit Location + Width  bit1=-470  base1=MSB of Input  bit0=0  base0=LSB of Input  dbl_ovrd=off  block_type=slice
  slice18 : xbsIndex_r4/Slice  nbits=10  boolean_output=off  mode=Upper Bit Location + Width  bit1=-460  base1=MSB of Input  bit0=0  base0=LSB of Input  dbl_ovrd=off  block_type=slice
  slice19 : xbsIndex_r4/Slice  nbits=10  boolean_output=off  mode=Upper Bit Location + Width  bit1=-450  base1=MSB of Input  bit0=0  base0=LSB of Input  dbl_ovrd=off  block_type=slice
  slice2 : xbsIndex_r4/Slice  nbits=10  boolean_output=off  mode=Upper Bit Location + Width  bit1=-620  base1=MSB of Input  bit0=0  base0=LSB of Input  dbl_ovrd=off  block_type=slice
  slice20 : xbsIndex_r4/Slice  nbits=10  boolean_output=off  mode=Upper Bit Location + Width  bit1=-440  base1=MSB of Input  bit0=0  base0=LSB of Input  dbl_ovrd=off  block_type=slice
  slice21 : xbsIndex_r4/Slice  nbits=10  boolean_output=off  mode=Upper Bit Location + Width  bit1=-430  base1=MSB of Input  bit0=0  base0=LSB of Input  dbl_ovrd=off  block_type=slice
  slice22 : xbsIndex_r4/Slice  nbits=10  boolean_output=off  mode=Upper Bit Location + Width  bit1=-420  base1=MSB of Input  bit0=0  base0=LSB of Input  dbl_ovrd=off  block_type=slice
  slice23 : xbsIndex_r4/Slice  nbits=10  boolean_output=off  mode=Upper Bit Location + Width  bit1=-410  base1=MSB of Input  bit0=0  base0=LSB of Input  dbl_ovrd=off  block_type=slice
  slice24 : xbsIndex_r4/Slice  nbits=10  boolean_output=off  mode=Upper Bit Location + Width  bit1=-400  base1=MSB of Input  bit0=0  base0=LSB of Input  dbl_ovrd=off  block_type=slice
  slice25 : xbsIndex_r4/Slice  nbits=10  boolean_output=off  mode=Upper Bit Location + Width  bit1=-390  base1=MSB of Input  bit0=0  base0=LSB of Input  dbl_ovrd=off  block_type=slice
  slice26 : xbsIndex_r4/Slice  nbits=10  boolean_output=off  mode=Upper Bit Location + Width  bit1=-380  base1=MSB of Input  bit0=0  base0=LSB of Input  dbl_ovrd=off  block_type=slice
  slice27 : xbsIndex_r4/Slice  nbits=10  boolean_output=off  mode=Upper Bit Location + Width  bit1=-370  base1=MSB of Input  bit0=0  base0=LSB of Input  dbl_ovrd=off  block_type=slice
  slice28 : xbsIndex_r4/Slice  nbits=10  boolean_output=off  mode=Upper Bit Location + Width  bit1=-360  base1=MSB of Input  bit0=0  base0=LSB of Input  dbl_ovrd=off  block_type=slice
  slice29 : xbsIndex_r4/Slice  nbits=10  boolean_output=off  mode=Upper Bit Location + Width  bit1=-350  base1=MSB of Input  bit0=0  base0=LSB of Input  dbl_ovrd=off  block_type=slice
  slice3 : xbsIndex_r4/Slice  nbits=10  boolean_output=off  mode=Upper Bit Location + Width  bit1=-610  base1=MSB of Input  bit0=0  base0=LSB of Input  dbl_ovrd=off  block_type=slice
  slice30 : xbsIndex_r4/Slice  nbits=10  boolean_output=off  mode=Upper Bit Location + Width  bit1=-340  base1=MSB of Input  bit0=0  base0=LSB of Input  dbl_ovrd=off  block_type=slice
  slice31 : xbsIndex_r4/Slice  nbits=10  boolean_output=off  mode=Upper Bit Location + Width  bit1=-330  base1=MSB of Input  bit0=0  base0=LSB of Input  dbl_ovrd=off  block_type=slice
  slice32 : xbsIndex_r4/Slice  nbits=10  boolean_output=off  mode=Upper Bit Location + Width  bit1=-320  base1=MSB of Input  bit0=0  base0=LSB of Input  dbl_ovrd=off  block_type=slice
  slice33 : xbsIndex_r4/Slice  nbits=10  boolean_output=off  mode=Upper Bit Location + Width  bit1=-310  base1=MSB of Input  bit0=0  base0=LSB of Input  dbl_ovrd=off  block_type=slice
  slice34 : xbsIndex_r4/Slice  nbits=10  boolean_output=off  mode=Upper Bit Location + Width  bit1=-300  base1=MSB of Input  bit0=0  base0=LSB of Input  dbl_ovrd=off  block_type=slice
  slice35 : xbsIndex_r4/Slice  nbits=10  boolean_output=off  mode=Upper Bit Location + Width  bit1=-290  base1=MSB of Input  bit0=0  base0=LSB of Input  dbl_ovrd=off  block_type=slice
  slice36 : xbsIndex_r4/Slice  nbits=10  boolean_output=off  mode=Upper Bit Location + Width  bit1=-280  base1=MSB of Input  bit0=0  base0=LSB of Input  dbl_ovrd=off  block_type=slice
  slice37 : xbsIndex_r4/Slice  nbits=10  boolean_output=off  mode=Upper Bit Location + Width  bit1=-270  base1=MSB of Input  bit0=0  base0=LSB of Input  dbl_ovrd=off  block_type=slice
  slice38 : xbsIndex_r4/Slice  nbits=10  boolean_output=off  mode=Upper Bit Location + Width  bit1=-260  base1=MSB of Input  bit0=0  base0=LSB of Input  dbl_ovrd=off  block_type=slice
  slice39 : xbsIndex_r4/Slice  nbits=10  boolean_output=off  mode=Upper Bit Location + Width  bit1=-250  base1=MSB of Input  bit0=0  base0=LSB of Input  dbl_ovrd=off  block_type=slice
  slice4 : xbsIndex_r4/Slice  nbits=10  boolean_output=off  mode=Upper Bit Location + Width  bit1=-600  base1=MSB of Input  bit0=0  base0=LSB of Input  dbl_ovrd=off  block_type=slice
  slice40 : xbsIndex_r4/Slice  nbits=10  boolean_output=off  mode=Upper Bit Location + Width  bit1=-240  base1=MSB of Input  bit0=0  base0=LSB of Input  dbl_ovrd=off  block_type=slice
  slice41 : xbsIndex_r4/Slice  nbits=10  boolean_output=off  mode=Upper Bit Location + Width  bit1=-230  base1=MSB of Input  bit0=0  base0=LSB of Input  dbl_ovrd=off  block_type=slice
  slice42 : xbsIndex_r4/Slice  nbits=10  boolean_output=off  mode=Upper Bit Location + Width  bit1=-220  base1=MSB of Input  bit0=0  base0=LSB of Input  dbl_ovrd=off  block_type=slice
  slice43 : xbsIndex_r4/Slice  nbits=10  boolean_output=off  mode=Upper Bit Location + Width  bit1=-210  base1=MSB of Input  bit0=0  base0=LSB of Input  dbl_ovrd=off  block_type=slice
  slice44 : xbsIndex_r4/Slice  nbits=10  boolean_output=off  mode=Upper Bit Location + Width  bit1=-200  base1=MSB of Input  bit0=0  base0=LSB of Input  dbl_ovrd=off  block_type=slice
  slice45 : xbsIndex_r4/Slice  nbits=10  boolean_output=off  mode=Upper Bit Location + Width  bit1=-190  base1=MSB of Input  bit0=0  base0=LSB of Input  dbl_ovrd=off  block_type=slice
  slice46 : xbsIndex_r4/Slice  nbits=10  boolean_output=off  mode=Upper Bit Location + Width  bit1=-180  base1=MSB of Input  bit0=0  base0=LSB of Input  dbl_ovrd=off  block_type=slice
  slice47 : xbsIndex_r4/Slice  nbits=10  boolean_output=off  mode=Upper Bit Location + Width  bit1=-170  base1=MSB of Input  bit0=0  base0=LSB of Input  dbl_ovrd=off  block_type=slice
  slice48 : xbsIndex_r4/Slice  nbits=10  boolean_output=off  mode=Upper Bit Location + Width  bit1=-160  base1=MSB of Input  bit0=0  base0=LSB of Input  dbl_ovrd=off  block_type=slice
  slice49 : xbsIndex_r4/Slice  nbits=10  boolean_output=off  mode=Upper Bit Location + Width  bit1=-150  base1=MSB of Input  bit0=0  base0=LSB of Input  dbl_ovrd=off  block_type=slice
  slice5 : xbsIndex_r4/Slice  nbits=10  boolean_output=off  mode=Upper Bit Location + Width  bit1=-590  base1=MSB of Input  bit0=0  base0=LSB of Input  dbl_ovrd=off  block_type=slice
  slice50 : xbsIndex_r4/Slice  nbits=10  boolean_output=off  mode=Upper Bit Location + Width  bit1=-140  base1=MSB of Input  bit0=0  base0=LSB of Input  dbl_ovrd=off  block_type=slice
  slice51 : xbsIndex_r4/Slice  nbits=10  boolean_output=off  mode=Upper Bit Location + Width  bit1=-130  base1=MSB of Input  bit0=0  base0=LSB of Input  dbl_ovrd=off  block_type=slice
  slice52 : xbsIndex_r4/Slice  nbits=10  boolean_output=off  mode=Upper Bit Location + Width  bit1=-120  base1=MSB of Input  bit0=0  base0=LSB of Input  dbl_ovrd=off  block_type=slice
  slice53 : xbsIndex_r4/Slice  nbits=10  boolean_output=off  mode=Upper Bit Location + Width  bit1=-110  base1=MSB of Input  bit0=0  base0=LSB of Input  dbl_ovrd=off  block_type=slice
  slice54 : xbsIndex_r4/Slice  nbits=10  boolean_output=off  mode=Upper Bit Location + Width  bit1=-100  base1=MSB of Input  bit0=0  base0=LSB of Input  dbl_ovrd=off  block_type=slice
  slice55 : xbsIndex_r4/Slice  nbits=10  boolean_output=off  mode=Upper Bit Location + Width  bit1=-90  base1=MSB of Input  bit0=0  base0=LSB of Input  dbl_ovrd=off  block_type=slice
  slice56 : xbsIndex_r4/Slice  nbits=10  boolean_output=off  mode=Upper Bit Location + Width  bit1=-80  base1=MSB of Input  bit0=0  base0=LSB of Input  dbl_ovrd=off  block_type=slice
  slice57 : xbsIndex_r4/Slice  nbits=10  boolean_output=off  mode=Upper Bit Location + Width  bit1=-70  base1=MSB of Input  bit0=0  base0=LSB of Input  dbl_ovrd=off  block_type=slice
  slice58 : xbsIndex_r4/Slice  nbits=10  boolean_output=off  mode=Upper Bit Location + Width  bit1=-60  base1=MSB of Input  bit0=0  base0=LSB of Input  dbl_ovrd=off  block_type=slice
  slice59 : xbsIndex_r4/Slice  nbits=10  boolean_output=off  mode=Upper Bit Location + Width  bit1=-50  base1=MSB of Input  bit0=0  base0=LSB of Input  dbl_ovrd=off  block_type=slice
  slice6 : xbsIndex_r4/Slice  nbits=10  boolean_output=off  mode=Upper Bit Location + Width  bit1=-580  base1=MSB of Input  bit0=0  base0=LSB of Input  dbl_ovrd=off  block_type=slice
  slice60 : xbsIndex_r4/Slice  nbits=10  boolean_output=off  mode=Upper Bit Location + Width  bit1=-40  base1=MSB of Input  bit0=0  base0=LSB of Input  dbl_ovrd=off  block_type=slice
  slice61 : xbsIndex_r4/Slice  nbits=10  boolean_output=off  mode=Upper Bit Location + Width  bit1=-30  base1=MSB of Input  bit0=0  base0=LSB of Input  dbl_ovrd=off  block_type=slice
  slice62 : xbsIndex_r4/Slice  nbits=10  boolean_output=off  mode=Upper Bit Location + Width  bit1=-20  base1=MSB of Input  bit0=0  base0=LSB of Input  dbl_ovrd=off  block_type=slice
  slice63 : xbsIndex_r4/Slice  nbits=10  boolean_output=off  mode=Upper Bit Location + Width  bit1=-10  base1=MSB of Input  bit0=0  base0=LSB of Input  dbl_ovrd=off  block_type=slice
  slice64 : xbsIndex_r4/Slice  nbits=10  boolean_output=off  mode=Upper Bit Location + Width  bit1=0  base1=MSB of Input  bit0=0  base0=LSB of Input  dbl_ovrd=off  block_type=slice
  slice7 : xbsIndex_r4/Slice  nbits=10  boolean_output=off  mode=Upper Bit Location + Width  bit1=-570  base1=MSB of Input  bit0=0  base0=LSB of Input  dbl_ovrd=off  block_type=slice
  slice8 : xbsIndex_r4/Slice  nbits=10  boolean_output=off  mode=Upper Bit Location + Width  bit1=-560  base1=MSB of Input  bit0=0  base0=LSB of Input  dbl_ovrd=off  block_type=slice
  slice9 : xbsIndex_r4/Slice  nbits=10  boolean_output=off  mode=Upper Bit Location + Width  bit1=-550  base1=MSB of Input  bit0=0  base0=LSB of Input  dbl_ovrd=off  block_type=slice
  msb_out64 : Outport
  out63 : Outport  Port=2
  out62 : Outport  Port=3
  out61 : Outport  Port=4
  out60 : Outport  Port=5
  out59 : Outport  Port=6
  out58 : Outport  Port=7
  out57 : Outport  Port=8
  out56 : Outport  Port=9
  out55 : Outport  Port=10
  out54 : Outport  Port=11
  out53 : Outport  Port=12
  out52 : Outport  Port=13
  out51 : Outport  Port=14
  out50 : Outport  Port=15
  out49 : Outport  Port=16
  out48 : Outport  Port=17
  out47 : Outport  Port=18
  out46 : Outport  Port=19
  out45 : Outport  Port=20
  out44 : Outport  Port=21
  out43 : Outport  Port=22
  out42 : Outport  Port=23
  out41 : Outport  Port=24
  out40 : Outport  Port=25
  out39 : Outport  Port=26
  out38 : Outport  Port=27
  out37 : Outport  Port=28
  out36 : Outport  Port=29
  out35 : Outport  Port=30
  out34 : Outport  Port=31
  out33 : Outport  Port=32
  out32 : Outport  Port=33
  out31 : Outport  Port=34
  out30 : Outport  Port=35
  out29 : Outport  Port=36
  out28 : Outport  Port=37
  out27 : Outport  Port=38
  out26 : Outport  Port=39
  out25 : Outport  Port=40
  out24 : Outport  Port=41
  out23 : Outport  Port=42
  out22 : Outport  Port=43
  out21 : Outport  Port=44
  out20 : Outport  Port=45
  out19 : Outport  Port=46
  out18 : Outport  Port=47
  out17 : Outport  Port=48
  out16 : Outport  Port=49
  out15 : Outport  Port=50
  out14 : Outport  Port=51
  out13 : Outport  Port=52
  out12 : Outport  Port=53
  out11 : Outport  Port=54
  out10 : Outport  Port=55
  out9 : Outport  Port=56
  out8 : Outport  Port=57
  out7 : Outport  Port=58
  out6 : Outport  Port=59
  out5 : Outport  Port=60
  out4 : Outport  Port=61
  out3 : Outport  Port=62
  out2 : Outport  Port=63
  lsb_out1 : Outport  Port=64
  wires:
  reinterpret1/1 -> lsb_out1/1
  slice1/1 -> reinterpret1/1
  reinterpret2/1 -> out2/1
  slice2/1 -> reinterpret2/1
  reinterpret3/1 -> out3/1
  slice3/1 -> reinterpret3/1
  reinterpret4/1 -> out4/1
  slice4/1 -> reinterpret4/1
  reinterpret5/1 -> out5/1
  slice5/1 -> reinterpret5/1
  reinterpret6/1 -> out6/1
  slice6/1 -> reinterpret6/1
  reinterpret7/1 -> out7/1
  slice7/1 -> reinterpret7/1
  reinterpret8/1 -> out8/1
  slice8/1 -> reinterpret8/1
  reinterpret9/1 -> out9/1
  slice9/1 -> reinterpret9/1
  reinterpret10/1 -> out10/1
  slice10/1 -> reinterpret10/1
  reinterpret11/1 -> out11/1
  slice11/1 -> reinterpret11/1
  reinterpret12/1 -> out12/1
  slice12/1 -> reinterpret12/1
  reinterpret13/1 -> out13/1
  slice13/1 -> reinterpret13/1
  reinterpret14/1 -> out14/1
  slice14/1 -> reinterpret14/1
  reinterpret15/1 -> out15/1
  slice15/1 -> reinterpret15/1
  reinterpret16/1 -> out16/1
  slice16/1 -> reinterpret16/1
  reinterpret17/1 -> out17/1
  slice17/1 -> reinterpret17/1
  reinterpret18/1 -> out18/1
  slice18/1 -> reinterpret18/1
  reinterpret19/1 -> out19/1
  slice19/1 -> reinterpret19/1
  reinterpret20/1 -> out20/1
  slice20/1 -> reinterpret20/1
  reinterpret21/1 -> out21/1
  slice21/1 -> reinterpret21/1
  reinterpret22/1 -> out22/1
  slice22/1 -> reinterpret22/1
  reinterpret23/1 -> out23/1
  slice23/1 -> reinterpret23/1
  reinterpret24/1 -> out24/1
  slice24/1 -> reinterpret24/1
  reinterpret25/1 -> out25/1
  slice25/1 -> reinterpret25/1
  reinterpret26/1 -> out26/1
  slice26/1 -> reinterpret26/1
  reinterpret27/1 -> out27/1
  slice27/1 -> reinterpret27/1
  reinterpret28/1 -> out28/1
  slice28/1 -> reinterpret28/1
  reinterpret29/1 -> out29/1
  slice29/1 -> reinterpret29/1
  reinterpret30/1 -> out30/1
  slice30/1 -> reinterpret30/1
  reinterpret31/1 -> out31/1
  slice31/1 -> reinterpret31/1
  reinterpret32/1 -> out32/1
  slice32/1 -> reinterpret32/1
  reinterpret33/1 -> out33/1
  slice33/1 -> reinterpret33/1
  reinterpret34/1 -> out34/1
  slice34/1 -> reinterpret34/1
  reinterpret35/1 -> out35/1
  slice35/1 -> reinterpret35/1
  reinterpret36/1 -> out36/1
  slice36/1 -> reinterpret36/1
  reinterpret37/1 -> out37/1
  slice37/1 -> reinterpret37/1
  reinterpret38/1 -> out38/1
  slice38/1 -> reinterpret38/1
  reinterpret39/1 -> out39/1
  slice39/1 -> reinterpret39/1
  reinterpret40/1 -> out40/1
  slice40/1 -> reinterpret40/1
  reinterpret41/1 -> out41/1
  slice41/1 -> reinterpret41/1
  reinterpret42/1 -> out42/1
  slice42/1 -> reinterpret42/1
  reinterpret43/1 -> out43/1
  slice43/1 -> reinterpret43/1
  reinterpret44/1 -> out44/1
  slice44/1 -> reinterpret44/1
  reinterpret45/1 -> out45/1
  slice45/1 -> reinterpret45/1
  reinterpret46/1 -> out46/1
  slice46/1 -> reinterpret46/1
  reinterpret47/1 -> out47/1
  slice47/1 -> reinterpret47/1
  reinterpret48/1 -> out48/1
  slice48/1 -> reinterpret48/1
  reinterpret49/1 -> out49/1
  slice49/1 -> reinterpret49/1
  reinterpret50/1 -> out50/1
  slice50/1 -> reinterpret50/1
  reinterpret51/1 -> out51/1
  slice51/1 -> reinterpret51/1
  reinterpret52/1 -> out52/1
  slice52/1 -> reinterpret52/1
  reinterpret53/1 -> out53/1
  slice53/1 -> reinterpret53/1
  reinterpret54/1 -> out54/1
  slice54/1 -> reinterpret54/1
  reinterpret55/1 -> out55/1
  slice55/1 -> reinterpret55/1
  reinterpret56/1 -> out56/1
  slice56/1 -> reinterpret56/1
  reinterpret57/1 -> out57/1
  slice57/1 -> reinterpret57/1
  reinterpret58/1 -> out58/1
  slice58/1 -> reinterpret58/1
  reinterpret59/1 -> out59/1
  slice59/1 -> reinterpret59/1
  reinterpret60/1 -> out60/1
  slice60/1 -> reinterpret60/1
  reinterpret61/1 -> out61/1
  slice61/1 -> reinterpret61/1
  reinterpret62/1 -> out62/1
  slice62/1 -> reinterpret62/1
  reinterpret63/1 -> out63/1
  slice63/1 -> reinterpret63/1
  reinterpret64/1 -> msb_out64/1
  slice64/1 -> reinterpret64/1
  bus_in/1 -> slice1/1, slice2/1, slice3/1, slice4/1, slice5/1, slice6/1, slice7/1, slice8/1, slice9/1, slice10/1, slice11/1, slice12/1, slice13/1, slice14/1, slice15/1, slice16/1, slice17/1, slice18/1, slice19/1, slice20/1, slice21/1, slice22/1, slice23/1, slice24/1, slice25/1, slice26/1, slice27/1, slice28/1, slice29/1, slice30/1, slice31/1, slice32/1, slice33/1, slice34/1, slice35/1, slice36/1, slice37/1, slice38/1, slice39/1, slice40/1, slice41/1, slice42/1, slice43/1, slice44/1, slice45/1, slice46/1, slice47/1, slice48/1, slice49/1, slice50/1, slice51/1, slice52/1, slice53/1, slice54/1, slice55/1, slice56/1, slice57/1, slice58/1, slice59/1, slice60/1, slice61/1, slice62/1, slice63/1, slice64/1
